simulink model "plaatb_m"  (Simulink 7.9)
settings: Solver=ode45  SolverMode=SingleTasking  StartTime=0.0  StopTime=999999  MaxStep=10  RelTol=1e-3  AbsTol=1e-3
values from neighbouring files (symbols this model uses):
  U = st_Varia('LongNames')    [plaatb_i.m]
  x0 = zeros(B.CStates+B.DStates,1)    [plaatb_i.m]    (also in plaatb_s.m = x0)
undefined symbols (not defined in the file or in its folder): B
settings Model: Creator=psross  LastModifiedBy=M.Sparnaaij
settings DataIOCC: LimitDataPoints=off  SaveOutput=off  SaveTime=off  SignalLoggingName=sigsOut
settings OptimizationCC: BooleanDataType=off
settings DebuggingCC: SaveWithParameterizedLinksMsg=none  SignalResolutionControl=TryResolveAllWithWarning  SolverPrmCheckMsg=none  MultiTaskDSMMsg=warning  MultiTaskCondExecSysMsg=none  FcnCallInpInsideContextMsg=Use local settings  StrictBusMsg=None
settings HardwareCC: TargetUnknown=on
settings RTWCC: IncludeERTFirstTime=on
settings GRTTargetCC: CombineOutputUpdateFcns=off  GRTInterface=on

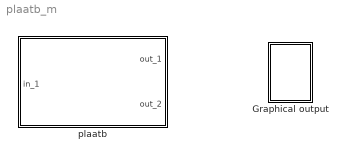
== system plaatb_m ==
  Graphical output : Subsystem
      settings: OpenFcn=plaatb_g
      mask Display:
      | plot(0,0,100,100,[80,20,20],[20,20,80],[80,69,60,52,45,39,33,28,24,20],[65,65,64,61,57,52,45,37,30,20])
      | disp('');
      | text(100,100,'plaatb', 'horizontalAlignment', 'right', 'verticalAlignment', 'top');
  plaatb : Subsystem  Description=This model calculates the aeration and degassifying with a weir aerator. The influent carbon dioxide concentration is calculated on the basis of the bicarbonate concentration, the pH, the EGV and the water temperature, so these parameters must always be filled out in the 'Water quality parameters' block.
      mask init:
      | filenaam='.\StimelaData\Weir_aerator.mat';
      | 
      | [Pn,Fn,Fext]=Fileprop(filenaam);
      | 
      | errstr = st_UniqName(filenaam,'filenaam=''','SubSystem','OpenFcn');
      | if errstr, error([errstr 'The filename "' filenaam '" is already in use. Choose a different filename.']), end
      | 
      | P = plaatb_p(filenaam);
      | [B,x0,U]=plaatb_i(filenaam);
      settings: OpenFcn=|
      | filenaam='.\StimelaData\Weir_aerator.mat';
      | st_ParameterInput('init',gcb,filenaam,'plaatb');
      mask Display:
      | plot(0,0,100,100,[20,80,80,20,20],[70,70,20,20,70],[80,90,90,90,9,9,20],[20,20,30,40,40,60,60],[80,20],[50,50],[11,10,8,6],[60,65,68,70],[15,14,12,10,6],[60,64,67,69,70],[78,78],[40,50],[84,83,82,80],[40,45,48,50],[87,86,84,80],[40,45,48,50],[64,64,67,67],[80,77,77,70],[64,73,73,70,70],[80,80,77,77,70],[70,67],[77,77])
      | disp('')
      | text(50,50,'plaatb', 'horizontalAlignment', 'center', 'verticalAlignment', 'middle');
      | text(50,0,Fn, 'horizontalAlignment', 'center', 'verticalAlignment', 'base');

== system plaatb_m/Graphical output ==
  note: plotten

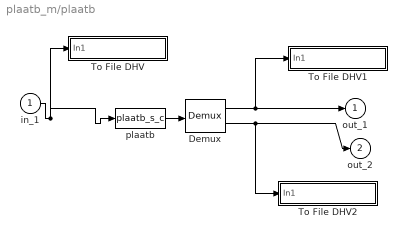
== system plaatb_m/plaatb ==
  in_1 : Inport
  Demux : Demux  Outputs=[U.Number B.Measurements]
  To File DHV : Subsystem  mask(To File DHV){naam=[filenaam(1:length(filenaam)-4) '_in.sti']}
      mask prompts: naam "Naam van bestand"
      mask init:
      | set_param([gcb '/To File'],'Filename',naam);
      mask Display: disp(naam)
  To File DHV1 : Subsystem  mask(To File DHV){naam=[filenaam(1:length(filenaam)-4) '_out.sti']}
      mask prompts: naam "Naam van bestand"
      mask init:
      | set_param([gcb '/To File'],'Filename',naam);
      mask Display: disp(naam)
  To File DHV2 : Subsystem  mask(To File DHV){naam=[filenaam(1:length(filenaam)-4) '_EM.sti']}
      mask prompts: naam "Naam van bestand"
      mask init:
      | set_param([gcb '/To File'],'Filename',naam);
      mask Display: disp(naam)
  plaatb : S-Function  FunctionName=plaatb_s_c  Parameters=B,x0,U,P  EnableBusSupport=off
  out_1 : Outport  InitialOutput=0
  out_2 : Outport  Port=2  InitialOutput=0
  wires:
  in_1/1 -> To File DHV/1(In1), plaatb/1
  Demux/2 -> To File DHV2/1(In1), out_2/1
  Demux/1 -> To File DHV1/1(In1), out_1/1
  plaatb/1 -> Demux/1

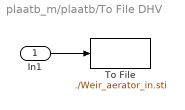
== system plaatb_m/plaatb/To File DHV ==
  In1 : Inport
  To File : ToFile  Filename=./Weir_aerator_in.sti  MatrixName=plaatbin
  wires:
  In1/1 -> To File/1

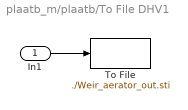
== system plaatb_m/plaatb/To File DHV1 ==
  In1 : Inport
  To File : ToFile  Filename=./Weir_aerator_out.sti  MatrixName=plaatbout
  wires:
  In1/1 -> To File/1

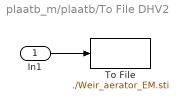
== system plaatb_m/plaatb/To File DHV2 ==
  In1 : Inport
  To File : ToFile  Filename=./Weir_aerator_EM.sti  MatrixName=plaatbEM
  wires:
  In1/1 -> To File/1
